simulink model "example531"  (R2017b)
settings: Solver=ode4  StartTime=0.0  StopTime=200  FixedStep=0.1  RelTol=1e-3
settings Model: Creator=GPL  LastModifiedBy=GPL

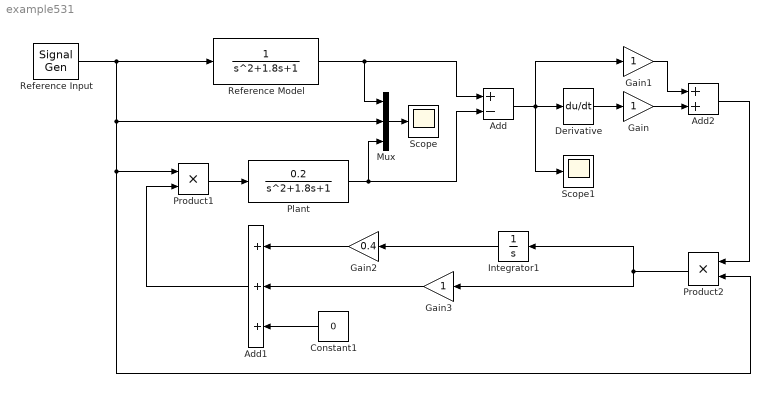
== system example531 ==
  Add : Sum  Inputs=+-
  Add1 : Sum  Inputs=+++
  Add2 : Sum
  Constant1 : Constant  Value=0
  Derivative : Derivative
  Gain : Gain
  Gain1 : Gain
  Gain2 : Gain  Gain=0.4
  Gain3 : Gain
  Integrator1 : Integrator
  Mux : Mux  Inputs=3
  Plant : TransferFcn  Numerator=[0.2]  Denominator=[1 1.8 1]
  Product1 : Product
  Product2 : Product
  Reference Input : SignalGenerator  WaveForm=square  Frequency=0.01
  Reference Model : TransferFcn  Denominator=[1 1.8 1]
  Scope : Scope
  Scope1 : Scope
  wires:
  Product1/1 -> Plant/1
  Reference Input/1 -> Mux/2, Product2/2, Product1/1, Reference Model/1
  Gain2/1 -> Add1/1
  Gain3/1 -> Add1/2
  Constant1/1 -> Add1/3
  Integrator1/1 -> Gain2/1
  Product2/1 -> Integrator1/1, Gain3/1
  Reference Model/1 -> Mux/1, Add/1
  Plant/1 -> Add/2, Mux/3
  Add/1 -> Scope1/1, Derivative/1, Gain1/1
  Derivative/1 -> Gain/1
  Gain/1 -> Add2/2
  Gain1/1 -> Add2/1
  Add2/1 -> Product2/1
  Add1/1 -> Product1/2
  Mux/1 -> Scope/1
